simulink model "PP_LE"  (R2024b)
settings: Solver=VariableStepAuto  StartTime=0.0  StopTime=20.0  RelTol=1e-3
values from neighbouring files (symbols this model uses):
  A = [ 0      1       0 ... (first row only)    [exam.m]    (also in exam2.m)
  B = [0; 0; 2/a(1)]    [exam.m]    (also in exam2.m; exam3.m = 0.01)
  C = eye(3)    [exam.m]    (also in exam2.m)
  D = Kp * (Td / Tvz)    [PID2PSDSquares.m]    (also in PID2PSDTrapezoids.m = Kp* (Td / Tvz); exam.m = 0; exam2.m = 0)
  disorder_times = [15, 16]    [exam.m]    (also in exam2.m; exam3.m = [12, 16]; exam4.m = [15, 25]; practical_exam_assignment3.m = [30, 40])
undefined symbols (not defined in the file or in its folder): K, N
settings Model: Creator=lukiq  LastModifiedBy=lukiq

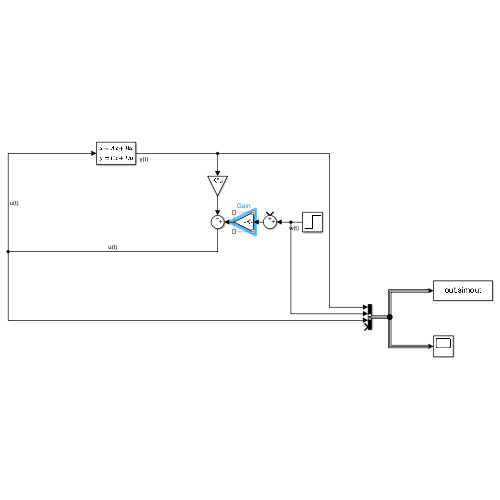
[thumbnail: Simulink's stored preview of the top-level diagram]
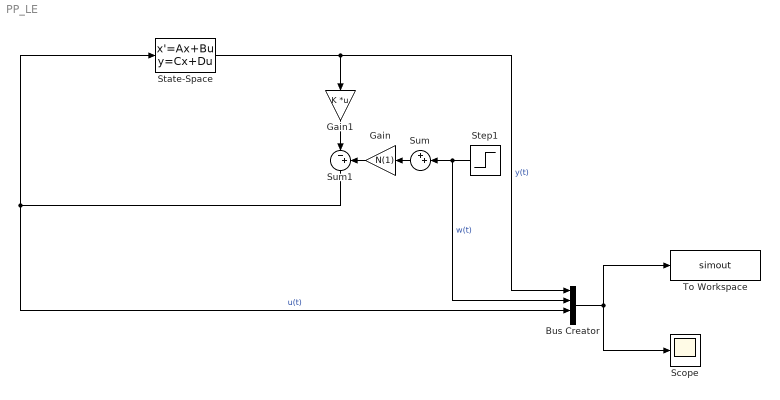
== system PP_LE ==
  Bus Creator : BusCreator  Inputs=4
  Gain : Gain  Gain=N(1)
  Gain1 : Gain  Gain=K  Multiplication=Matrix(K*u)
  Scope : Scope
  State-Space : StateSpace  A=A  B=B  C=C  D=D  InitialCondition=0
  Step1 : Step  Time=disorder_times(1)  SampleTime=0
  Sum : Sum  Inputs=++|
  Sum1 : Sum  Inputs=|-+
  To Workspace : ToWorkspace  VariableName=simout  SaveFormat=Timeseries  SampleTime=-1
  wires:
  Sum1/1 -> State-Space/1, Bus Creator/3  "u(t)"
  Bus Creator/1 -> Scope/1, To Workspace/1
  Gain1/1 -> Sum1/1
  Step1/1 -> Bus Creator/2, Sum/2  "w(t)"
  Gain/1 -> Sum1/2
  Sum/1 -> Gain/1
  State-Space/1 -> Gain1/1, Bus Creator/1  "y(t)"
